simulink model "sim_lab7_disturbances"  (R2025b)
settings: Solver=ode5  StartTime=0.0  StopTime=5*T  FixedStep=1  RelTol=1e-3
model workspace (MAT data in the model file):
  Pnull = Simulink.Parameter
  Pnull.Value = Simulink.data.Expression
  Pnull.Value.ExpressionString = "zeros(3,1)"
  Pnull.Complexity = 'real'
  Pnull.Dimensions = -1
  Pnull.DataType = 'auto'
  rho_albedo_medio = Simulink.Parameter
  rho_albedo_medio.Value = 0.3
  rho_albedo_medio.Complexity = 'real'
  rho_albedo_medio.Dimensions = [1 1]
  rho_albedo_medio.DataType = 'auto'
values from neighbouring files (symbols this model uses):
  Aree = zeros(10,1)    [SCRIPT_SAD_DEMO.m]    (also in lab_7.m)
  c = astroConstants(5)*1e3    [SCRIPT_SAD_DEMO.m]    (also in lab_7.m)
  eps_E = deg2rad(astroConstants(63))    [SCRIPT_SAD_DEMO.m]    (also in lab_7.m)
  F_e = 1358    [SCRIPT_SAD_DEMO.m]    (also in lab_7.m)
  g0_1 = -29404.8e-9    (= -2.94048e-05)    [lab_7.m]
  g1_1 = -1450.9e-9    (= -1.4509e-06)    [lab_7.m]
  h1_1 = 4652.5e-9    (= 4.6525e-06)    [lab_7.m]
  j_B = [0.01; 0.05; 0.01]    [SCRIPT_SAD_DEMO.m]    (also in lab_7.m)
  J_depl = [100.9, 0, 0;           0, 25.1, 0;           0, 0, 91.6]*1e-2    [SCRIPT_SAD_DEMO.m]    (also in lab_7.m)
  kep = [a,e,incl,raan,w,theta]    [SCRIPT_SAD_DEMO.m]    (also in lab_7.m)
  mu = astroConstants(13)    [SCRIPT_SAD_DEMO.m]    (also in lab_7.m)
  n = sqrt( (mu/ (a)^3))    [SCRIPT_SAD_DEMO.m]    (also in lab_7.m = sqrt((mu/ ((a/1000)^3))))
  n_sun = 2*pi/T_sun    (= 1.99238499086e-07)    [SCRIPT_SAD_DEMO.m]    (also in lab_7.m)
  Nmat = [ ... (first row only)    [SCRIPT_SAD_DEMO.m]    (also in lab_7.m)
  r_sun = 1*ua    [SCRIPT_SAD_DEMO.m]    (also in lab_7.m)
  Re = astroConstants(23)    [SCRIPT_SAD_DEMO.m]    (also in lab_7.m)
  rf = [ ... (first row only)    [SCRIPT_SAD_DEMO.m]    (also in lab_7.m)
  rhod = 0.1*ones(10,1)    [SCRIPT_SAD_DEMO.m]    (also in lab_7.m)
  rhos = zeros(10,1)    [SCRIPT_SAD_DEMO.m]    (also in lab_7.m)
  theta = 0    [SCRIPT_SAD_DEMO.m]    (also in lab_7.m)
  w_E = deg2rad(15.04)/3600    [SCRIPT_SAD_DEMO.m]    (also in lab_7.m)
undefined symbols (not defined in the file or in its folder): SRP
libraries: LIBRARY_SAD x16, matrix_library x15
settings Model: Creator=fabio  LastModifiedBy=utente

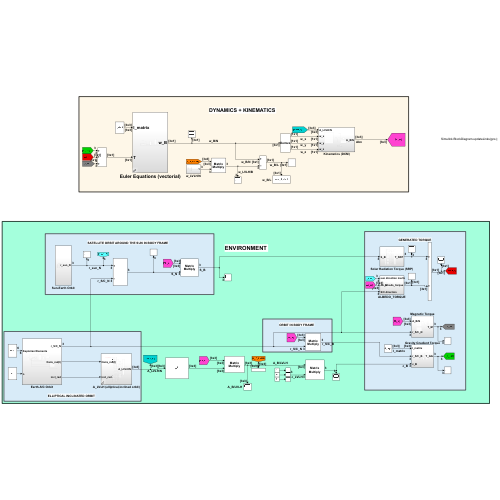
[thumbnail: Simulink's stored preview of the top-level diagram]
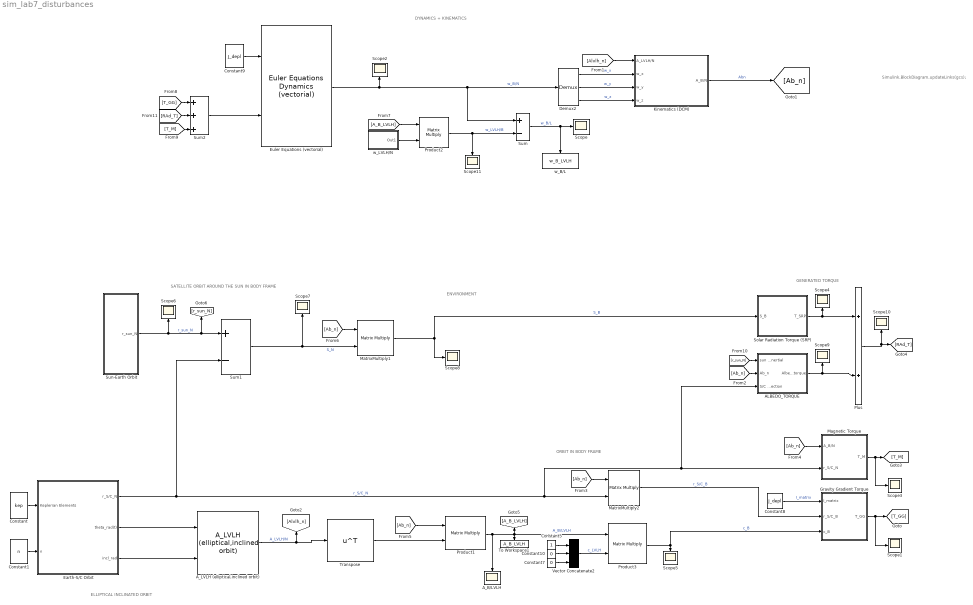
== system sim_lab7_disturbances ==
  note: Simulink.BlockDiagram.updateLinks(gcs);
  note: ORBIT IN BODY FRAME
  note: SATELLITE ORBIT AROUND THE SUN IN BODY FRAME
  note: GENERATED TORQUE
  note: ELLIPTICAL INCLINATED ORBIT
  note: ENVIRONMENT
  note: DYNAMICS + KINEMATICS
  ALBEDO_TORQUE : Subsystem
  A_B/LVLH : Scope
      settings: ActiveDisplayYMinimum=-0.55999388120508109  ActiveDisplayYMaximum=1.1733326534672313
  A_LVLH (elliptical,inclined orbit) : LIBRARY_SAD/A_LVLH (elliptical,inclined orbit)  SystemSampleTime=-1  VariantActivationTime=update diagram  EmptyChoice=off  PassThrough=off  PassThroughVariantControl=(default)  EmptyChoiceVariantControl=(default)  AllowFlexibleInterface=on  Latency=0  AutoFrameSizeCalculation=off
  Constant : Constant  Value=kep
  Constant1 : Constant  Value=n
  Constant10 : Constant  Value=0
  Constant5 : Constant
  Constant7 : Constant  Value=0
  Constant8 : Constant  Value=J_depl
  Constant9 : Constant  Value=J_depl
  Demux2 : Demux  Outputs=3
      settings: DisplayOption=none
  Earth-S/C Orbit : Subsystem
  Euler Equations (vectorial) : LIBRARY_SAD/Euler Equations Dynamics (vectorial)  SystemSampleTime=-1  VariantActivationTime=update diagram  EmptyChoice=off  PassThrough=off  PassThroughVariantControl=(default)  EmptyChoiceVariantControl=(default)  AllowFlexibleInterface=on  Latency=0  AutoFrameSizeCalculation=off
  Gravity Gradient Torque : Subsystem
  Kinematics (DCM) : Subsystem
  Magnetic Torque : Subsystem
  MatrixMultiply1 : Product  Multiplication=Matrix(*)
  MatrixMultiply2 : Product  Multiplication=Matrix(*)
  Plus : Sum
  Product1 : Product  Multiplication=Matrix(*)
  Product2 : Product  Multiplication=Matrix(*)
  Product3 : Product  Multiplication=Matrix(*)
  Scope{,1..11} (12 alike) : Scope
      Scope settings: ActiveDisplayYMinimum=-1.5011598737710617E-6  ActiveDisplayYMaximum=2.8262196534247165E-6
      Scope1 settings: DataLoggingVariableName=ScopeData3
      Scope10 settings: ActiveDisplayYMinimum=-1  ActiveDisplayYMaximum=1  DataLoggingVariableName=ScopeData27
      Scope11 settings: ActiveDisplayYMinimum=-1  ActiveDisplayYMaximum=1  DataLoggingVariableName=ScopeData21
      Scope2 settings: ActiveDisplayYMinimum=-0.00010343063306164844  ActiveDisplayYMaximum=0.00093087569755483622  DataLoggingVariableName=ScopeData2
      Scope3 settings: ActiveDisplayYMinimum=-1.6923991885641683E-6  ActiveDisplayYMaximum=1.7159675183701099E-6  DataLoggingVariableName=ScopeData4
      Scope4 settings: ActiveDisplayYMinimum=-4.3087224502121108E-24  ActiveDisplayYMaximum=4.3087224502121108E-24  DataLoggingVariableName=ScopeData16
      Scope5 settings: ActiveDisplayYMinimum=-0.55998948749949928  ActiveDisplayYMaximum=1.1733321652777222  DataLoggingVariableName=ScopeData20
      Scope6 settings: ActiveDisplayYMinimum=-1  ActiveDisplayYMaximum=1  DataLoggingVariableName=ScopeData6
      Scope7 settings: ActiveDisplayYMinimum=-1  ActiveDisplayYMaximum=1  DataLoggingVariableName=ScopeData7
      Scope8 settings: DataLoggingVariableName=ScopeData8
      Scope9 settings: ActiveDisplayYMinimum=-9.2718061255302776E-25  ActiveDisplayYMaximum=9.2718061255302776E-25  DataLoggingVariableName=ScopeData26
  Solar Radiation Torque (SRP) : Subsystem
  Sum : Sum  Inputs=+-
  Sum1 : Sum  Inputs=+-
  Sum2 : Sum  Inputs=+++
  Sun-Earth Orbit : Subsystem
  To Workspace1 : ToWorkspace  VariableName=A_B_LVLH  SampleTime=-1
  Transpose : Math  Operator=transpose
  Vector Concatenate2 : Concatenate  NumInputs=3
  w_B/L : ToWorkspace  VariableName=w_B_LVLH  SampleTime=-1
  w_LVLH/N : Subsystem
  wires:
  Euler Equations (vectorial)/1 -> Demux2/1, Sum/1, Scope2/1  "w_B/N"
  Demux2/3 -> Kinematics (DCM)/4(w_z)  "w_z"
  Product2/1 -> Scope11/1, Sum/2  "w_LVLH/B"
  Transpose/1 -> Product1/2
  Demux2/1 -> Kinematics (DCM)/2(w_x)  "w_x"
  A_LVLH (elliptical,inclined orbit)/1 -> [Alvlh_n], Transpose/1  "A_LVLH/N"
  Sum1/1 -> Scope7/1, MatrixMultiply1/2  "S_N"
  Constant/1 -> Earth-S/C Orbit/1(Keplerian Elements)
  Earth-S/C Orbit/3(incl_rad) -> A_LVLH (elliptical,inclined orbit)/2
  Product3/1 -> Gravity Gradient Torque/3(c_B), Scope5/1  "c_B"
  Constant8/1 -> Gravity Gradient Torque/1(I_matrix)  "I_matrix"
  Product1/1 -> Product3/1, [A_B_LVLH], To Workspace1/1, A_B/LVLH/1  "A_B/LVLH"
  Earth-S/C Orbit/2(theta_rad(t)) -> A_LVLH (elliptical,inclined orbit)/1
  MatrixMultiply2/1 -> Gravity Gradient Torque/2(r_S/C_B)  "r_S/C_B"
  Vector Concatenate2/1 -> Product3/2  "c_LVLH"
  Constant1/1 -> Earth-S/C Orbit/2(n)
  Constant5/1 -> Vector Concatenate2/1
  Sum2/1 -> Euler Equations (vectorial)/2
  Earth-S/C Orbit/1(r_S/C_N) -> Sum1/2, MatrixMultiply2/2, ALBEDO_TORQUE/3(S/C direction), Magnetic Torque/2(r_S/C_N)  "r_S/C_N"
  Constant10/1 -> Vector Concatenate2/2
  Constant7/1 -> Vector Concatenate2/3
  Sum/1 -> w_B/L/1, Scope/1  "w_B/L"
  Demux2/2 -> Kinematics (DCM)/3(w_y)  "w_y"
  Sun-Earth Orbit/1(r_sun_N) -> Scope6/1, Sum1/1, [r_sun_N]  "r_sun_N"
  MatrixMultiply1/1 -> Scope8/1, Solar Radiation Torque (SRP)/1(S_B)  "S_B"
  Kinematics (DCM)/1(A_B/N) -> [Ab_n]  "Abn"
  Constant9/1 -> Euler Equations (vectorial)/1
  [Ab_n] -> MatrixMultiply1/1
  [Ab_n] -> Magnetic Torque/1(A_B/N)
  [Ab_n] -> MatrixMultiply2/1
  [Ab_n] -> Product1/1
  [Alvlh_n] -> Kinematics (DCM)/1(A_LVLH/N)
  [A_B_LVLH] -> Product2/1
  Gravity Gradient Torque/1(T_GG) -> Scope1/1, [T_GG]
  Magnetic Torque/1(T_M) -> Scope3/1, [T_M]
  Solar Radiation Torque (SRP)/1(T_SRP) -> Plus/1, Scope4/1
  [RAd_T] -> Sum2/2
  [T_GG] -> Sum2/1
  [T_M] -> Sum2/3
  w_LVLH/N/1(Out1) -> Product2/2
  [r_sun_N] -> ALBEDO_TORQUE/1(sun direction inertial)
  [Ab_n] -> ALBEDO_TORQUE/2(Ab_n)
  ALBEDO_TORQUE/1(Albedo_torque) -> Scope9/1, Plus/2
  Plus/1 -> Scope10/1, [RAd_T]

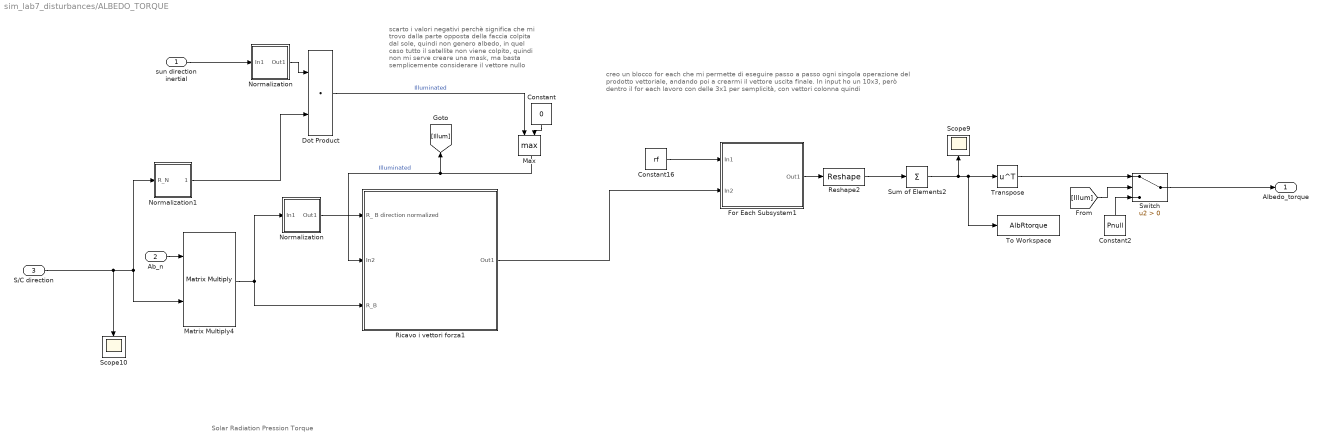
== system sim_lab7_disturbances/ALBEDO_TORQUE ==
  note: Solar Radiation Pression Torque
  note: creo un blocco for each che mi permette di eseguire passo a passo ogni singola operazione del prodotto vettoriale, andando poi a crearmi il vettore uscita finale. In input ho un 10x3, però dentro il for each lavoro con delle 3x1 per semplicità, con vettori colonna quindi
  note: scarto i valori negativi perchè significa che mi trovo dalla parte opposta della faccia colpita dal sole, quindi non genero albedo, in quel caso tutto il satellite non viene colpito, quindi non mi serve creare una mask, ma basta semplicemente considerare il vettore nullo
  sun direction inertial : Inport
  Ab_n : Inport  Port=2
  S/C direction : Inport  Port=3
  Constant : Constant  Value=0
  Constant16 : Constant  Value=rf
  Constant2 : Constant  Value=Pnull
  Dot Product : DotProduct  OutDataTypeStr=Inherit: Inherit via internal rule
  For Each Subsystem1 : Subsystem  TreatAsAtomicUnit=on
  Matrix Multiply4 : Product  Multiplication=Matrix(*)
  Max : MinMax  Function=max  Inputs=2
  Normalization : Subsystem
  "Normalization " : Subsystem
  Normalization1 : Subsystem
  Reshape2 : Reshape  OutputDimensionality=Customize  OutputDimensions=[10 3]
  Ricavo i vettori forza1 : Subsystem
  Scope10 : Scope
      settings: ActiveDisplayYMinimum=-8805.2567998384475  ActiveDisplayYMaximum=8127.929464306656  DataLoggingVariableName=ScopeData17
  Scope9 : Scope
      settings: ActiveDisplayYMinimum=-9.2718061255302776E-25  ActiveDisplayYMaximum=2.6543612251060555E-24  DataLoggingVariableName=ScopeData25
  Sum of Elements2 : Sum  Inputs=+  CollapseMode=Specified dimension
  Switch : Switch  Criteria=u2 > Threshold  SaturateOnIntegerOverflow=off  InputSameDT=off
  To Workspace : ToWorkspace  VariableName=AlbRtorque  SampleTime=-1
  Transpose : Math  Operator=transpose
  Albedo_torque : Outport
  wires:
  Sum of Elements2/1 -> Transpose/1, To Workspace/1, Scope9/1
  Matrix Multiply4/1 -> Normalization/1(In1), Ricavo i vettori forza1/3(R_B)
  Normalization1/1(Out1) -> Dot Product/2
  Ricavo i vettori forza1/1(Out1) -> For Each Subsystem1/2(In2)
  For Each Subsystem1/1(Out1) -> Reshape2/1
  S/C direction/1 -> Scope10/1, Matrix Multiply4/2, Normalization1/1(R_N)
  "Normalization "/1(Out1) -> Dot Product/1
  Constant16/1 -> For Each Subsystem1/1(In1)
  Normalization/1(Out1) -> Ricavo i vettori forza1/1(" R_ B direction normalized")
  Dot Product/1 -> Max/1  "Illuminated"
  Ab_n/1 -> Matrix Multiply4/1
  sun direction inertial/1 -> "Normalization "/1(In1)
  Constant2/1 -> Switch/3
  Reshape2/1 -> Sum of Elements2/1
  Constant/1 -> Max/2
  Transpose/1 -> Switch/1
  Switch/1 -> Albedo_torque/1
  Max/1 -> Ricavo i vettori forza1/2(In2), [Illum]  "Illuminated"
  [Illum] -> Switch/2

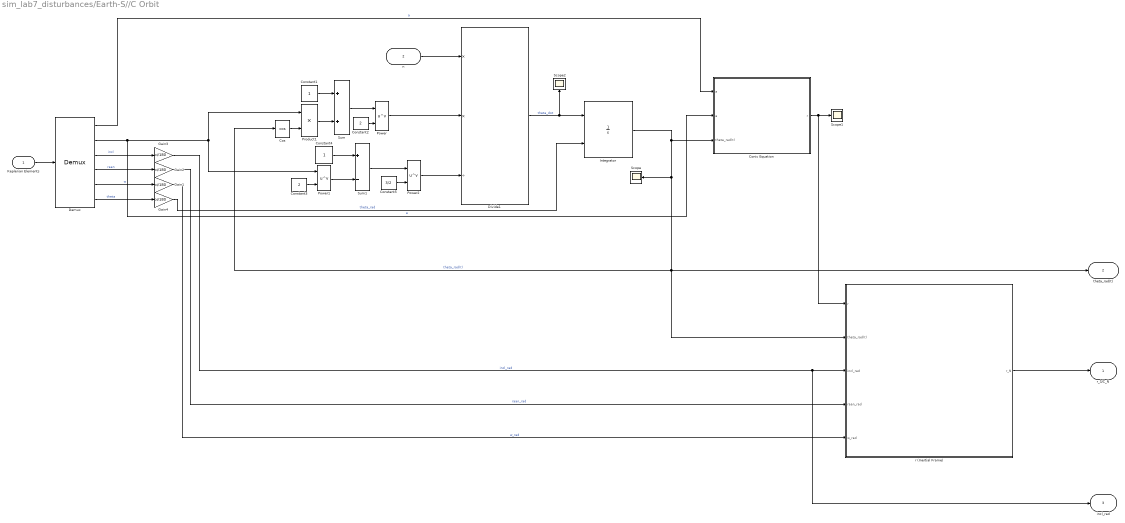
== system sim_lab7_disturbances/Earth-S//C Orbit ==
  Keplerian Elements : Inport
  n : Inport  Port=2
  Conic Equation : Subsystem
  Constant1 : Constant
  Constant2 : Constant  Value=2
  Constant3 : Constant  Value=2
  Constant4 : Constant
  Constant5 : Constant  Value=3/2
  Cos : Trigonometry  Operator=cos
  Demux : Demux  Outputs=6
      settings: DisplayOption=none
  Divide1 : Product  Inputs=**/
  Gain{1..4} (4 alike) : Gain  Gain=pi/180
  Integrator : Integrator  InitialConditionSource=external  InitialCondition=theta  WrapState=on  WrappedStateUpperValue=2*pi  WrappedStateLowerValue=0
  Power : Math  Operator=pow
  Power1 : Math  Operator=pow
  Power2 : Math  Operator=pow
  Product1 : Product
  Scope : Scope
      settings: ActiveDisplayYMinimum=-0.785387370168924  ActiveDisplayYMaximum=7.0684863315203179  DataLoggingVariableName=ScopeData22
  Scope1 : Scope
      settings: ActiveDisplayYMinimum=6287.5500000061184  ActiveDisplayYMaximum=10412.44999994494  DataLoggingVariableName=ScopeData23
  Scope2 : Scope
      settings: ActiveDisplayYMinimum=0.00072744506449318766  ActiveDisplayYMaximum=0.00092744506449318775  DataLoggingVariableName=ScopeData24
  Sum : Sum
  Sum1 : Sum  Inputs=+-
  r (Inertial Frame) : Subsystem
  r_S/C_N : Outport
  theta_rad(t) : Outport  Port=2
  incl_rad : Outport  Port=3
  wires:
  Keplerian Elements/1 -> Demux/1
  Demux/1 -> Conic Equation/1(a)  "a"
  Demux/2 -> Conic Equation/2(e), Product1/1, Power1/1  "e"
  Demux/3 -> Gain3/1  "incl"
  Demux/4 -> Gain2/1  "raan"
  Demux/5 -> Gain1/1  "w"
  Demux/6 -> Gain4/1  "theta"
  Constant1/1 -> Sum/1
  Cos/1 -> Product1/2
  Product1/1 -> Sum/2
  Sum/1 -> Power/1
  Constant2/1 -> Power/2
  Power/1 -> Divide1/2
  Constant3/1 -> Power1/2
  Power1/1 -> Sum1/2
  Constant4/1 -> Sum1/1
  Constant5/1 -> Power2/2
  Sum1/1 -> Power2/1
  Power2/1 -> Divide1/3
  Divide1/1 -> Scope2/1, Integrator/1  "theta_dot"
  Integrator/1 -> Scope/1, Cos/1, r (Inertial Frame)/2(theta_rad(t)), theta_rad(t)/1, Conic Equation/3(theta_rad(t))  "theta_rad(t)"
  Conic Equation/1(r) -> r (Inertial Frame)/1(r), Scope1/1
  Gain3/1 -> incl_rad/1, r (Inertial Frame)/3(incl_rad)  "incl_rad"
  Gain2/1 -> r (Inertial Frame)/4(raan_rad)  "raan_rad"
  Gain1/1 -> r (Inertial Frame)/5(w_rad)  "w_rad"
  r (Inertial Frame)/1(r_N) -> r_S/C_N/1
  n/1 -> Divide1/1
  Gain4/1 -> Integrator/2  "theta_rad"

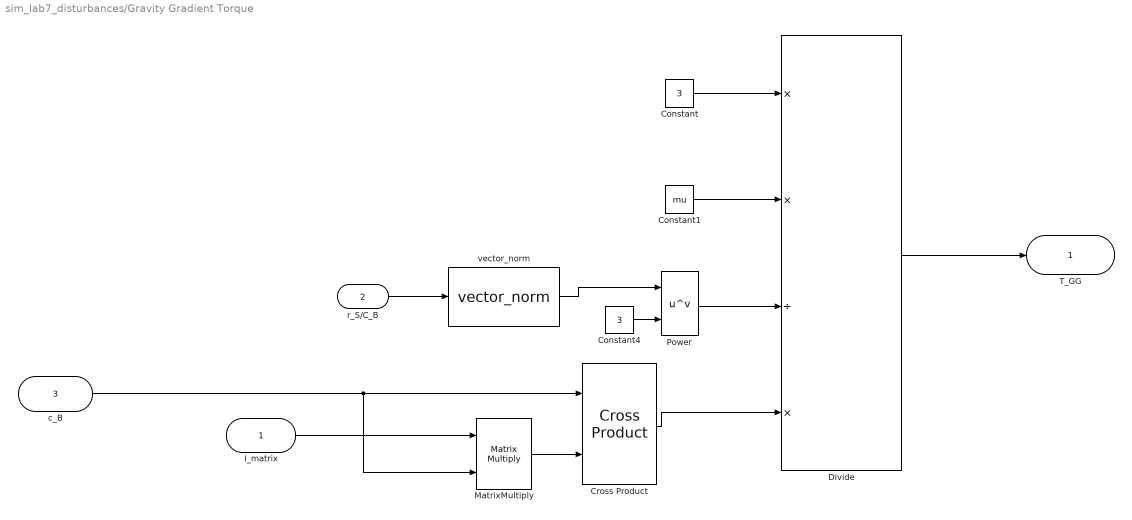
== system sim_lab7_disturbances/Gravity Gradient Torque ==
  I_matrix : Inport
  r_S/C_B : Inport  Port=2
  c_B : Inport  Port=3
  Constant : Constant  Value=3
  Constant1 : Constant  Value=mu
  Constant4 : Constant  Value=3
  Cross Product : matrix_library/Cross Product
  Divide : Product  Inputs=**/*
  MatrixMultiply : Product  Multiplication=Matrix(*)
  Power : Math  Operator=pow
  vector_norm : LIBRARY_SAD/vector_norm  SystemSampleTime=-1  VariantActivationTime=update diagram  EmptyChoice=off  PassThrough=off  PassThroughVariantControl=(default)  EmptyChoiceVariantControl=(default)  AllowFlexibleInterface=on  Latency=0  AutoFrameSizeCalculation=off
  T_GG : Outport
  wires:
  r_S/C_B/1 -> vector_norm/1
  Constant4/1 -> Power/2
  Constant/1 -> Divide/1
  Constant1/1 -> Divide/2
  Power/1 -> Divide/3
  I_matrix/1 -> MatrixMultiply/1
  c_B/1 -> MatrixMultiply/2, Cross Product/1
  MatrixMultiply/1 -> Cross Product/2
  Cross Product/1 -> Divide/4
  Divide/1 -> T_GG/1
  vector_norm/1 -> Power/1

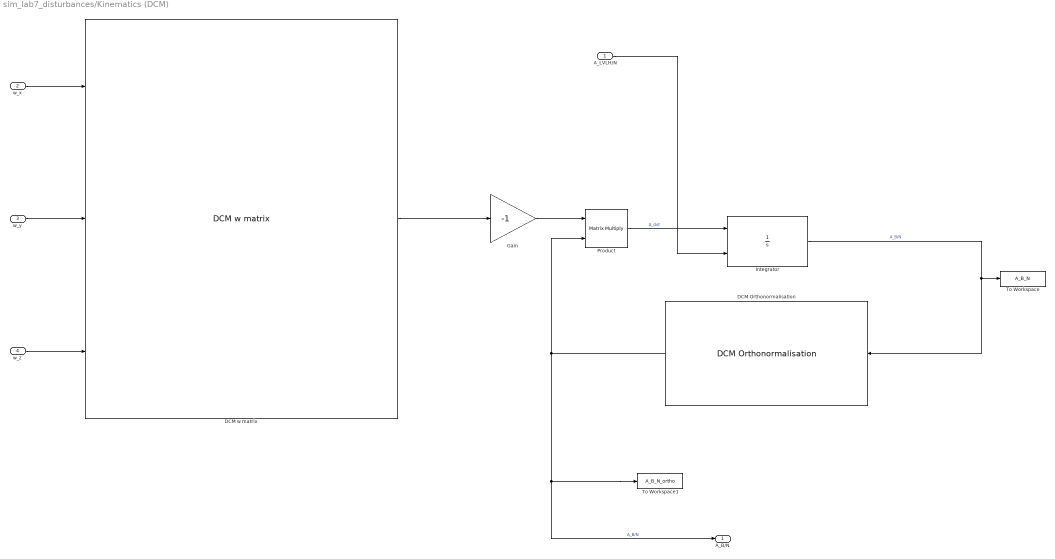
== system sim_lab7_disturbances/Kinematics (DCM) ==
  A_LVLH/N : Inport
  w_x : Inport  Port=2
  w_y : Inport  Port=3
  w_z : Inport  Port=4
  DCM Orthonormalisation : LIBRARY_SAD/DCM Orthonormalisation  SystemSampleTime=-1  VariantActivationTime=update diagram  EmptyChoice=off  PassThrough=off  PassThroughVariantControl=(default)  EmptyChoiceVariantControl=(default)  AllowFlexibleInterface=on  Latency=0  AutoFrameSizeCalculation=off
  DCM w matrix : LIBRARY_SAD/DCM w matrix  SystemSampleTime=-1  VariantActivationTime=update diagram  EmptyChoice=off  PassThrough=off  PassThroughVariantControl=(default)  EmptyChoiceVariantControl=(default)  AllowFlexibleInterface=on  Latency=0  AutoFrameSizeCalculation=off
  Gain : Gain  Gain=-1
  Integrator : Integrator  InitialConditionSource=external
  Product : Product  Multiplication=Matrix(*)
  To Workspace : ToWorkspace  VariableName=A_B_N  SampleTime=-1
  To Workspace1 : ToWorkspace  VariableName=A_B_N_ortho  SampleTime=-1
  A_B/N : Outport
  wires:
  A_LVLH/N/1 -> Integrator/2
  w_y/1 -> DCM w matrix/2
  w_z/1 -> DCM w matrix/3
  Integrator/1 -> To Workspace/1, DCM Orthonormalisation/1  "A_B/N"
  Product/1 -> Integrator/1  "A_dot"
  DCM w matrix/1 -> Gain/1
  w_x/1 -> DCM w matrix/1
  Gain/1 -> Product/1
  DCM Orthonormalisation/1 -> To Workspace1/1, A_B/N/1, Product/2  "A_B/N"

== system sim_lab7_disturbances/Magnetic Torque ==
  A_B/N : Inport
  r_S/C_N : Inport  Port=2
  B_N (IGRF Gauss Model - Order N) : Subsystem  Commented=on
  B_N (Simple Dipole Model) : Subsystem
  Constant : Constant  Value=j_B
  Cross Product : matrix_library/Cross Product
  MatrixMultiply : Product  Multiplication=Matrix(*)
  Scope : Scope
      settings: ActiveDisplayYMinimum=-1  ActiveDisplayYMaximum=1  DataLoggingVariableName=ScopeData5
  T_M : Outport
  wires:
  r_S/C_N/1 -> B_N (Simple Dipole Model)/1(r_S/C_N)
  B_N (Simple Dipole Model)/1(B_N) -> MatrixMultiply/2
  A_B/N/1 -> MatrixMultiply/1
  MatrixMultiply/1 -> Scope/1, Cross Product/2  "B_B"
  Constant/1 -> Cross Product/1
  Cross Product/1 -> T_M/1

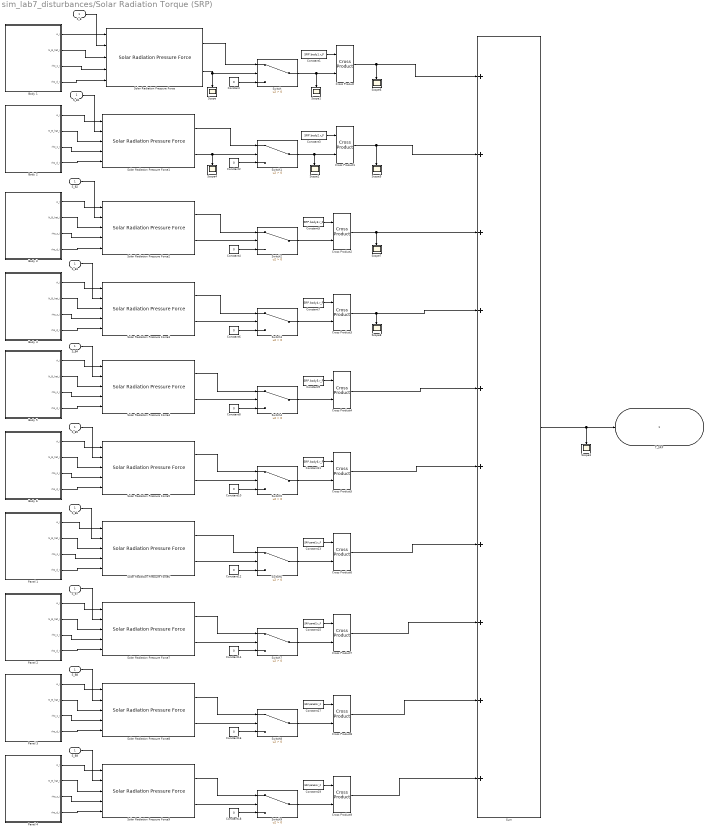
== system sim_lab7_disturbances/Solar Radiation Torque (SRP) ==
  S_B : Inport
  Body 1 : Subsystem
  Body 2 : Subsystem
  Body 3 : Subsystem
  Body 4 : Subsystem
  Body 5 : Subsystem
  Body 6 : Subsystem
  Constant{,2,4,6,8,10,12,14,16,18} (10 alike) : Constant  Value=0
  Constant1 : Constant  Value=SRP.body1.r_F
  Constant11 : Constant  Value=SRP.body6.r_F
  Constant13 : Constant  Value=SRP.panel1.r_F
  Constant15 : Constant  Value=SRP.panel2.r_F
  Constant17 : Constant  Value=SRP.panel3.r_F
  Constant19 : Constant  Value=SRP.panel4.r_F
  Constant3 : Constant  Value=SRP.body2.r_F
  Constant5 : Constant  Value=SRP.body3.r_F
  Constant7 : Constant  Value=SRP.body4.r_F
  Constant9 : Constant  Value=SRP.body5.r_F
  Cross Product{,1..9} (10 alike) : matrix_library/Cross Product
  Panel 1 : Subsystem
  Panel 2 : Subsystem
  Panel 3 : Subsystem
  Panel 4 : Subsystem
  S_B{1..9} (9 alike) : InportShadow
  Scope{,1..8} (9 alike) : Scope
      Scope settings: ActiveDisplayYMinimum=-1  ActiveDisplayYMaximum=1  DataLoggingVariableName=ScopeData9
      Scope1 settings: ActiveDisplayYMinimum=-1  ActiveDisplayYMaximum=1  DataLoggingVariableName=ScopeData10
      Scope2 settings: ActiveDisplayYMinimum=-1  ActiveDisplayYMaximum=1  DataLoggingVariableName=ScopeData11
      Scope3 settings: ActiveDisplayYMinimum=-5.1359030627651383E-25  ActiveDisplayYMaximum=9.2718061255302776E-25  DataLoggingVariableName=ScopeData12
      Scope4 settings: ActiveDisplayYMinimum=-1  ActiveDisplayYMaximum=1  DataLoggingVariableName=ScopeData13
      Scope5 settings: ActiveDisplayYMinimum=-1  ActiveDisplayYMaximum=1  DataLoggingVariableName=ScopeData14
      Scope6 settings: ActiveDisplayYMinimum=-1  ActiveDisplayYMaximum=1  DataLoggingVariableName=ScopeData15
      Scope7 settings: ActiveDisplayYMinimum=-1  ActiveDisplayYMaximum=1  DataLoggingVariableName=ScopeData18
      Scope8 settings: ActiveDisplayYMinimum=-1  ActiveDisplayYMaximum=1  DataLoggingVariableName=ScopeData19
  Solar Radiation Pressure Force : LIBRARY_SAD/Solar Radiation Pressure Force  SystemSampleTime=-1  VariantActivationTime=update diagram  EmptyChoice=off  PassThrough=off  PassThroughVariantControl=(default)  EmptyChoiceVariantControl=(default)  AllowFlexibleInterface=on  Latency=0  AutoFrameSizeCalculation=off
      link override vector_norm: SourceBlock=LIBRARY_SAD/vector_norm
  Solar Radiation Pressure Force1 : LIBRARY_SAD/Solar Radiation Pressure Force  SystemSampleTime=-1  VariantActivationTime=update diagram  EmptyChoice=off  PassThrough=off  PassThroughVariantControl=(default)  EmptyChoiceVariantControl=(default)  AllowFlexibleInterface=on  Latency=0  AutoFrameSizeCalculation=off
      link override vector_norm: SourceBlock=LIBRARY_SAD/vector_norm
  Solar Radiation Pressure Force2 : LIBRARY_SAD/Solar Radiation Pressure Force  SystemSampleTime=-1  VariantActivationTime=update diagram  EmptyChoice=off  PassThrough=off  PassThroughVariantControl=(default)  EmptyChoiceVariantControl=(default)  AllowFlexibleInterface=on  Latency=0  AutoFrameSizeCalculation=off
      link override vector_norm: SourceBlock=LIBRARY_SAD/vector_norm
  Solar Radiation Pressure Force3 : LIBRARY_SAD/Solar Radiation Pressure Force  SystemSampleTime=-1  VariantActivationTime=update diagram  EmptyChoice=off  PassThrough=off  PassThroughVariantControl=(default)  EmptyChoiceVariantControl=(default)  AllowFlexibleInterface=on  Latency=0  AutoFrameSizeCalculation=off
      link override vector_norm: SourceBlock=LIBRARY_SAD/vector_norm
  Solar Radiation Pressure Force4 : LIBRARY_SAD/Solar Radiation Pressure Force  SystemSampleTime=-1  VariantActivationTime=update diagram  EmptyChoice=off  PassThrough=off  PassThroughVariantControl=(default)  EmptyChoiceVariantControl=(default)  AllowFlexibleInterface=on  Latency=0  AutoFrameSizeCalculation=off
      link override vector_norm: SourceBlock=LIBRARY_SAD/vector_norm
  Solar Radiation Pressure Force5 : LIBRARY_SAD/Solar Radiation Pressure Force  SystemSampleTime=-1  VariantActivationTime=update diagram  EmptyChoice=off  PassThrough=off  PassThroughVariantControl=(default)  EmptyChoiceVariantControl=(default)  AllowFlexibleInterface=on  Latency=0  AutoFrameSizeCalculation=off
      link override vector_norm: SourceBlock=LIBRARY_SAD/vector_norm
  Solar Radiation Pressure Force6 : LIBRARY_SAD/Solar Radiation Pressure Force  SystemSampleTime=-1  VariantActivationTime=update diagram  EmptyChoice=off  PassThrough=off  PassThroughVariantControl=(default)  EmptyChoiceVariantControl=(default)  AllowFlexibleInterface=on  Latency=0  AutoFrameSizeCalculation=off
      link override vector_norm: SourceBlock=LIBRARY_SAD/vector_norm
  Solar Radiation Pressure Force7 : LIBRARY_SAD/Solar Radiation Pressure Force  SystemSampleTime=-1  VariantActivationTime=update diagram  EmptyChoice=off  PassThrough=off  PassThroughVariantControl=(default)  EmptyChoiceVariantControl=(default)  AllowFlexibleInterface=on  Latency=0  AutoFrameSizeCalculation=off
      link override vector_norm: SourceBlock=LIBRARY_SAD/vector_norm
  Solar Radiation Pressure Force8 : LIBRARY_SAD/Solar Radiation Pressure Force  SystemSampleTime=-1  VariantActivationTime=update diagram  EmptyChoice=off  PassThrough=off  PassThroughVariantControl=(default)  EmptyChoiceVariantControl=(default)  AllowFlexibleInterface=on  Latency=0  AutoFrameSizeCalculation=off
      link override vector_norm: SourceBlock=LIBRARY_SAD/vector_norm
  Solar Radiation Pressure Force9 : LIBRARY_SAD/Solar Radiation Pressure Force  SystemSampleTime=-1  VariantActivationTime=update diagram  EmptyChoice=off  PassThrough=off  PassThroughVariantControl=(default)  EmptyChoiceVariantControl=(default)  AllowFlexibleInterface=on  Latency=0  AutoFrameSizeCalculation=off
      link override vector_norm: SourceBlock=LIBRARY_SAD/vector_norm
  Sum : Sum  Inputs=++++++++++
  Switch{,1..9} (10 alike) : Switch  Criteria=u2 > Threshold  SaturateOnIntegerOverflow=off  InputSameDT=off
  T_SRP : Outport
  wires:
  S_B/1 -> Solar Radiation Pressure Force/2
  Body 1/1(A_i) -> Solar Radiation Pressure Force/1
  Body 1/2(N_B_hat_i) -> Solar Radiation Pressure Force/3
  Body 1/3(rho_s_i) -> Solar Radiation Pressure Force/4
  Body 1/4(rho_d_i) -> Solar Radiation Pressure Force/5
  Solar Radiation Pressure Force/1 -> Switch/1
  Solar Radiation Pressure Force/2 -> Scope/1, Switch/2
  Body 2/4(rho_d_i) -> Solar Radiation Pressure Force1/5
  Body 2/3(rho_s_i) -> Solar Radiation Pressure Force1/4
  Body 2/2(N_B_hat_i) -> Solar Radiation Pressure Force1/3
  Body 2/1(A_i) -> Solar Radiation Pressure Force1/1
  S_B1/1 -> Solar Radiation Pressure Force1/2
  S_B2/1 -> Solar Radiation Pressure Force2/2
  Body 3/1(A_i) -> Solar Radiation Pressure Force2/1
  Body 3/2(N_B_hat_i) -> Solar Radiation Pressure Force2/3
  Body 3/3(rho_s_i) -> Solar Radiation Pressure Force2/4
  Body 3/4(rho_d_i) -> Solar Radiation Pressure Force2/5
  Body 4/4(rho_d_i) -> Solar Radiation Pressure Force3/5
  Body 4/3(rho_s_i) -> Solar Radiation Pressure Force3/4
  Body 4/2(N_B_hat_i) -> Solar Radiation Pressure Force3/3
  Body 4/1(A_i) -> Solar Radiation Pressure Force3/1
  S_B3/1 -> Solar Radiation Pressure Force3/2
  S_B4/1 -> Solar Radiation Pressure Force4/2
  Body 5/1(A_i) -> Solar Radiation Pressure Force4/1
  Body 5/2(N_B_hat_i) -> Solar Radiation Pressure Force4/3
  Body 5/3(rho_s_i) -> Solar Radiation Pressure Force4/4
  Body 5/4(rho_d_i) -> Solar Radiation Pressure Force4/5
  Body 6/4(rho_d_i) -> Solar Radiation Pressure Force5/5
  Body 6/3(rho_s_i) -> Solar Radiation Pressure Force5/4
  Body 6/2(N_B_hat_i) -> Solar Radiation Pressure Force5/3
  Body 6/1(A_i) -> Solar Radiation Pressure Force5/1
  S_B5/1 -> Solar Radiation Pressure Force5/2
  S_B6/1 -> Solar Radiation Pressure Force6/2
  Panel 1/1(A_i) -> Solar Radiation Pressure Force6/1
  Panel 1/2(N_B_hat_i) -> Solar Radiation Pressure Force6/3
  Panel 1/3(rho_s_i) -> Solar Radiation Pressure Force6/4
  Panel 1/4(rho_d_i) -> Solar Radiation Pressure Force6/5
  Panel 2/4(rho_d_i) -> Solar Radiation Pressure Force7/5
  Panel 2/3(rho_s_i) -> Solar Radiation Pressure Force7/4
  Panel 2/2(N_B_hat_i) -> Solar Radiation Pressure Force7/3
  Panel 2/1(A_i) -> Solar Radiation Pressure Force7/1
  S_B7/1 -> Solar Radiation Pressure Force7/2
  S_B8/1 -> Solar Radiation Pressure Force8/2
  Panel 3/1(A_i) -> Solar Radiation Pressure Force8/1
  Panel 3/2(N_B_hat_i) -> Solar Radiation Pressure Force8/3
  Panel 3/3(rho_s_i) -> Solar Radiation Pressure Force8/4
  Panel 3/4(rho_d_i) -> Solar Radiation Pressure Force8/5
  Panel 4/4(rho_d_i) -> Solar Radiation Pressure Force9/5
  Panel 4/3(rho_s_i) -> Solar Radiation Pressure Force9/4
  Panel 4/2(N_B_hat_i) -> Solar Radiation Pressure Force9/3
  Panel 4/1(A_i) -> Solar Radiation Pressure Force9/1
  S_B9/1 -> Solar Radiation Pressure Force9/2
  Constant/1 -> Switch/3
  Switch/1 -> Scope1/1, Cross Product/2
  Constant1/1 -> Cross Product/1
  Cross Product/1 -> Scope6/1, Sum/1
  Cross Product1/1 -> Sum/2, Scope5/1
  Constant3/1 -> Cross Product1/1
  Switch1/1 -> Scope2/1, Cross Product1/2
  Constant2/1 -> Switch1/3
  Solar Radiation Pressure Force1/2 -> Scope4/1, Switch1/2
  Solar Radiation Pressure Force1/1 -> Switch1/1
  Solar Radiation Pressure Force2/1 -> Switch2/1
  Solar Radiation Pressure Force2/2 -> Switch2/2
  Constant4/1 -> Switch2/3
  Switch2/1 -> Cross Product2/2
  Constant5/1 -> Cross Product2/1
  Cross Product2/1 -> Scope7/1, Sum/3
  Cross Product3/1 -> Scope8/1, Sum/4
  Constant7/1 -> Cross Product3/1
  Switch3/1 -> Cross Product3/2
  Constant6/1 -> Switch3/3
  Solar Radiation Pressure Force3/2 -> Switch3/2
  Solar Radiation Pressure Force3/1 -> Switch3/1
  Solar Radiation Pressure Force4/1 -> Switch4/1
  Solar Radiation Pressure Force4/2 -> Switch4/2
  Constant8/1 -> Switch4/3
  Switch4/1 -> Cross Product4/2
  Constant9/1 -> Cross Product4/1
  Cross Product4/1 -> Sum/5
  Cross Product5/1 -> Sum/6
  Constant11/1 -> Cross Product5/1
  Switch5/1 -> Cross Product5/2
  Constant10/1 -> Switch5/3
  Solar Radiation Pressure Force5/2 -> Switch5/2
  Solar Radiation Pressure Force5/1 -> Switch5/1
  Solar Radiation Pressure Force6/1 -> Switch6/1
  Solar Radiation Pressure Force6/2 -> Switch6/2
  Constant12/1 -> Switch6/3
  Switch6/1 -> Cross Product6/2
  Constant13/1 -> Cross Product6/1
  Cross Product6/1 -> Sum/7
  Cross Product7/1 -> Sum/8
  Constant15/1 -> Cross Product7/1
  Switch7/1 -> Cross Product7/2
  Constant14/1 -> Switch7/3
  Solar Radiation Pressure Force7/2 -> Switch7/2
  Solar Radiation Pressure Force7/1 -> Switch7/1
  Solar Radiation Pressure Force8/1 -> Switch8/1
  Solar Radiation Pressure Force8/2 -> Switch8/2
  Constant16/1 -> Switch8/3
  Switch8/1 -> Cross Product8/2
  Constant17/1 -> Cross Product8/1
  Cross Product8/1 -> Sum/9
  Cross Product9/1 -> Sum/10
  Constant19/1 -> Cross Product9/1
  Switch9/1 -> Cross Product9/2
  Constant18/1 -> Switch9/3
  Solar Radiation Pressure Force9/2 -> Switch9/2
  Solar Radiation Pressure Force9/1 -> Switch9/1
  Sum/1 -> Scope3/1, T_SRP/1

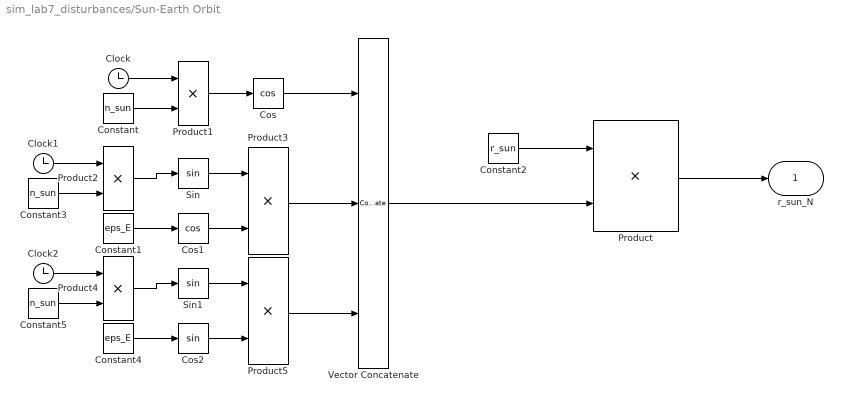
== system sim_lab7_disturbances/Sun-Earth Orbit ==
  Clock : Clock
  Clock1 : Clock
  Clock2 : Clock
  Constant : Constant  Value=n_sun
  Constant1 : Constant  Value=eps_E
  Constant2 : Constant  Value=r_sun
  Constant3 : Constant  Value=n_sun
  Constant4 : Constant  Value=eps_E
  Constant5 : Constant  Value=n_sun
  Cos : Trigonometry  Operator=cos
  Cos1 : Trigonometry  Operator=cos
  Cos2 : Trigonometry
  Product{,1..5} (6 alike) : Product
  Sin : Trigonometry
  Sin1 : Trigonometry
  Vector Concatenate : Concatenate  NumInputs=3
  r_sun_N : Outport
  wires:
  Constant2/1 -> Product/1
  Clock/1 -> Product1/1
  Constant/1 -> Product1/2
  Product1/1 -> Cos/1
  Cos/1 -> Vector Concatenate/1
  Product2/1 -> Sin/1
  Constant3/1 -> Product2/2
  Clock1/1 -> Product2/1
  Sin/1 -> Product3/1
  Constant1/1 -> Cos1/1
  Product3/1 -> Vector Concatenate/2
  Cos1/1 -> Product3/2
  Cos2/1 -> Product5/2
  Product5/1 -> Vector Concatenate/3
  Constant4/1 -> Cos2/1
  Sin1/1 -> Product5/1
  Clock2/1 -> Product4/1
  Constant5/1 -> Product4/2
  Product4/1 -> Sin1/1
  Vector Concatenate/1 -> Product/2
  Product/1 -> r_sun_N/1

== system sim_lab7_disturbances/w_LVLH//N ==
  Constant2 : Constant  Value=0
  Constant3 : Constant  Value=0
  Constant4 : Constant  Value=n
  Vector Concatenate1 : Concatenate  NumInputs=3
  Out1 : Outport
  wires:
  Vector Concatenate1/1 -> Out1/1  "w_LVLH/N"
  Constant2/1 -> Vector Concatenate1/1
  Constant3/1 -> Vector Concatenate1/2
  Constant4/1 -> Vector Concatenate1/3

== system sim_lab7_disturbances/ALBEDO_TORQUE/For Each Subsystem1 ==
  note: nelle proprietà lascio direttamente così almeno posso processare una alla volta le singole righe e colonne sia in dimension che in width
  In1 : Inport  Partition=on  PartitionDimension=1  PartitionWidth=1  PartitionOffset=0
  In2 : Inport  Port=2  Partition=on  PartitionDimension=1  PartitionWidth=1  PartitionOffset=0
  Cross Product : matrix_library/Cross Product
  For Each : ForEach  DisableCoverage=on
  Signal Specification : SignalSpecification  Dimensions=[1 3]
  Transpose : Math  Operator=transpose
  Transpose1 : Math  Operator=transpose
  Transpose2 : Math  Operator=transpose
  Out1 : Outport  ConcatenationDimension=1
  wires:
  In2/1 -> Transpose/1  "Rfi"
  In1/1 -> Transpose1/1  "Fi"
  Transpose/1 -> Cross Product/1
  Transpose1/1 -> Cross Product/2
  Cross Product/1 -> Transpose2/1
  Transpose2/1 -> Signal Specification/1
  Signal Specification/1 -> Out1/1

== system sim_lab7_disturbances/ALBEDO_TORQUE/Normalization ==
  In1 : Inport
  Divide : Product  Inputs=*/
  Dot Product : DotProduct  OutDataTypeStr=Inherit: Inherit via internal rule
  Sqrt : Sqrt
  Out1 : Outport
  wires:
  Dot Product/1 -> Sqrt/1
  In1/1 -> Divide/1, Dot Product/2, Dot Product/1
  Divide/1 -> Out1/1
  Sqrt/1 -> Divide/2

== system sim_lab7_disturbances/ALBEDO_TORQUE/Normalization  ==
  In1 : Inport
  Divide : Product  Inputs=*/
  Dot Product : DotProduct  OutDataTypeStr=Inherit: Inherit via internal rule
  Sqrt : Sqrt
  Out1 : Outport
  wires:
  Dot Product/1 -> Sqrt/1
  In1/1 -> Divide/1, Dot Product/2, Dot Product/1
  Divide/1 -> Out1/1
  Sqrt/1 -> Divide/2

== system sim_lab7_disturbances/ALBEDO_TORQUE/Normalization1 ==
  R_N : Inport
  Divide : Product  Inputs=*/
  Dot Product : DotProduct  OutDataTypeStr=Inherit: Inherit via internal rule
  Sqrt : Sqrt
  Out1 : Outport
  wires:
  Dot Product/1 -> Sqrt/1
  R_N/1 -> Divide/1, Dot Product/2, Dot Product/1
  Divide/1 -> Out1/1
  Sqrt/1 -> Divide/2

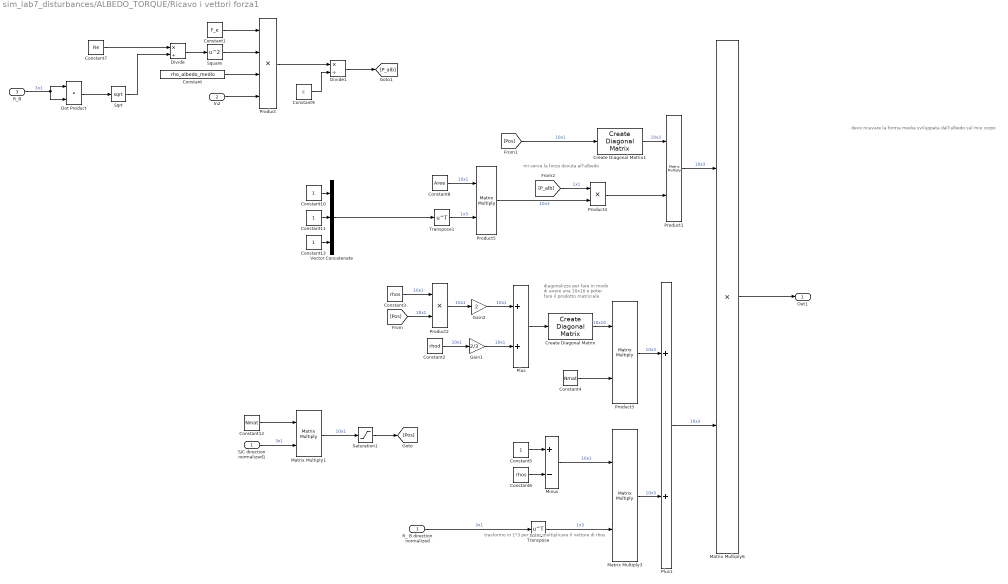
== system sim_lab7_disturbances/ALBEDO_TORQUE/Ricavo i vettori forza1 ==
  note: devo ricavare la forma media sviluppata dall'albedo sul mio corpo
  note: mi serve la forza dovuta all'albedo
  note: diagonalizzo per fare in modo di avere una 10x10 e poter fare il prodotto matriciale
  note: trasformo in 1*3 per poter moltiplicare il vettore di rhos
  " R_ B direction normalized" : Inport
  In2 : Inport  Port=2
  R_B : Inport  Port=3
  Constant : Constant  Value=rho_albedo_medio
  Constant1 : Constant  Value=F_e
  Constant{5,10..11,13} (4 alike) : Constant
  Constant12 : Constant  Value=Nmat
  Constant2 : Constant  Value=rhod
  Constant3 : Constant  Value=rhos
  Constant4 : Constant  Value=Nmat
  Constant6 : Constant  Value=rhos
  Constant7 : Constant  Value=Re
  Constant8 : Constant  Value=Aree
  Constant9 : Constant  Value=c
  Create Diagonal Matrix : matrix_library/Create Diagonal Matrix
      settings: LibrarySourceBlock=|
      | simulink/Matrix
      | Operations/Create Diagonal
      | Matrix
  Create Diagonal Matrix1 : matrix_library/Create Diagonal Matrix
      settings: LibrarySourceBlock=|
      | simulink/Matrix
      | Operations/Create Diagonal
      | Matrix
  Divide : Product  Inputs=*/
  Divide1 : Product  Inputs=*/
  Dot Product : DotProduct  OutDataTypeStr=Inherit: Inherit via internal rule
  Gain1 : Gain  Gain=2/3
  Gain2 : Gain  Gain=2
  Matrix Multiply1 : Product  Multiplication=Matrix(*)
  Matrix Multiply3 : Product  Multiplication=Matrix(*)
  Matrix Multiply6 : Product
  Minus : Sum  Inputs=+-
  Plus : Sum
  Plus1 : Sum
  Product : Product  Inputs=4
  Product1 : Product  Multiplication=Matrix(*)
  Product2 : Product
  Product3 : Product  Multiplication=Matrix(*)
  Product4 : Product
  Product5 : Product  Multiplication=Matrix(*)
  S/C direction normalized1 : InportShadow
  Saturation1 : Saturate  UpperLimit=inf  LowerLimit=0
  Sqrt : Sqrt
  Square : Math  Operator=square
  Transpose : Math  Operator=transpose
  Transpose1 : Math  Operator=transpose
  Vector Concatenate : Concatenate  NumInputs=3
  Out1 : Outport
  wires:
  Gain1/1 -> Plus/2  "10x1"
  Plus1/1 -> Matrix Multiply6/2  "10x3"
  Product3/1 -> Plus1/1  "10x3"
  Constant4/1 -> Product3/2
  Product2/1 -> Gain2/1  "10x1"
  Constant2/1 -> Gain1/1  "10x1"
  Constant6/1 -> Minus/2
  Constant3/1 -> Product2/1  "10x1"
  Product1/1 -> Matrix Multiply6/1  "10x3"
  Gain2/1 -> Plus/1  "10x1"
  " R_ B direction normalized"/1 -> Transpose/1  "3x1"
  Matrix Multiply3/1 -> Plus1/2  "10x3"
  Constant5/1 -> Minus/1
  Matrix Multiply6/1 -> Out1/1
  [Pos] -> Create Diagonal Matrix1/1  "10x1"
  Matrix Multiply1/1 -> Saturation1/1  "10x1"
  Constant12/1 -> Matrix Multiply1/1
  Minus/1 -> Matrix Multiply3/1  "10x1"
  Transpose/1 -> Matrix Multiply3/2  "1x3"
  Saturation1/1 -> [Pos]
  [Pos] -> Product2/2  "10x1"
  Plus/1 -> Create Diagonal Matrix/1
  Constant13/1 -> Vector Concatenate/3
  Constant10/1 -> Vector Concatenate/1
  Constant11/1 -> Vector Concatenate/2
  Vector Concatenate/1 -> Transpose1/1
  Create Diagonal Matrix/1 -> Product3/1  "10x10"
  Transpose1/1 -> Product5/2  "1x3"
  Constant8/1 -> Product5/1  "10x1"
  Product5/1 -> Product4/2  "10x3"
  Create Diagonal Matrix1/1 -> Product1/1  "10x3"
  Product4/1 -> Product1/2
  S/C direction normalized1/1 -> Matrix Multiply1/2  "3x1"
  Constant7/1 -> Divide/1
  Divide/1 -> Square/1
  Constant1/1 -> Product/1
  Square/1 -> Product/2
  Constant/1 -> Product/3
  In2/1 -> Product/4
  Product/1 -> Divide1/1
  Constant9/1 -> Divide1/2
  Divide1/1 -> [P_alb]
  [P_alb] -> Product4/1  "1x1"
  Sqrt/1 -> Divide/2
  R_B/1 -> Dot Product/1, Dot Product/2  "3x1"
  Dot Product/1 -> Sqrt/1

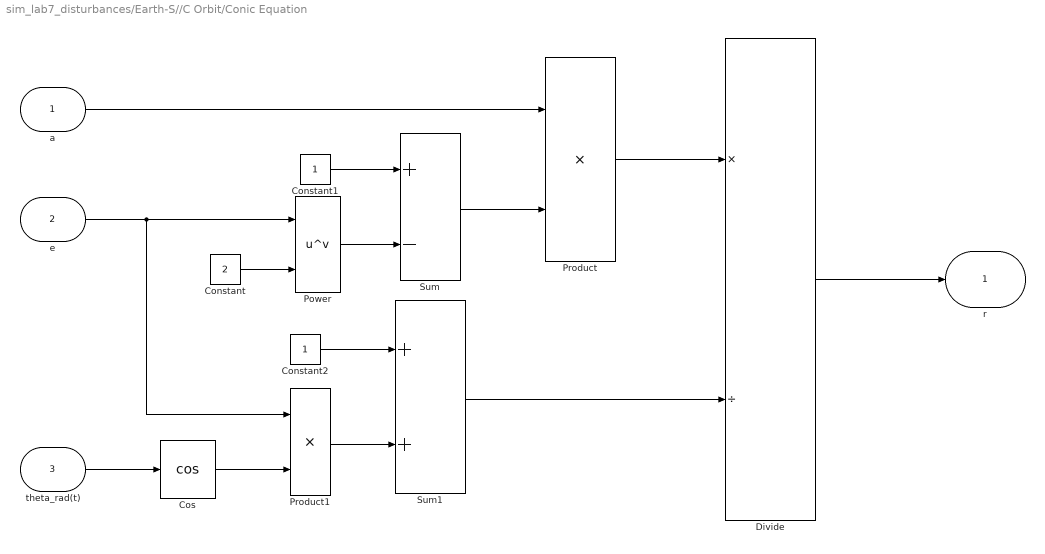
== system sim_lab7_disturbances/Earth-S//C Orbit/Conic Equation ==
  a : Inport
  e : Inport  Port=2
  theta_rad(t) : Inport  Port=3
  Constant : Constant  Value=2
  Constant1 : Constant
  Constant2 : Constant
  Cos : Trigonometry  Operator=cos
  Divide : Product  Inputs=*/
  Power : Math  Operator=pow
  Product : Product
  Product1 : Product
  Sum : Sum  Inputs=+-
  Sum1 : Sum
  r : Outport
  wires:
  a/1 -> Product/1
  e/1 -> Product1/1, Power/1
  Constant/1 -> Power/2
  Power/1 -> Sum/2
  Constant1/1 -> Sum/1
  Sum/1 -> Product/2
  Product/1 -> Divide/1
  Divide/1 -> r/1
  Constant2/1 -> Sum1/1
  theta_rad(t)/1 -> Cos/1
  Cos/1 -> Product1/2
  Product1/1 -> Sum1/2
  Sum1/1 -> Divide/2

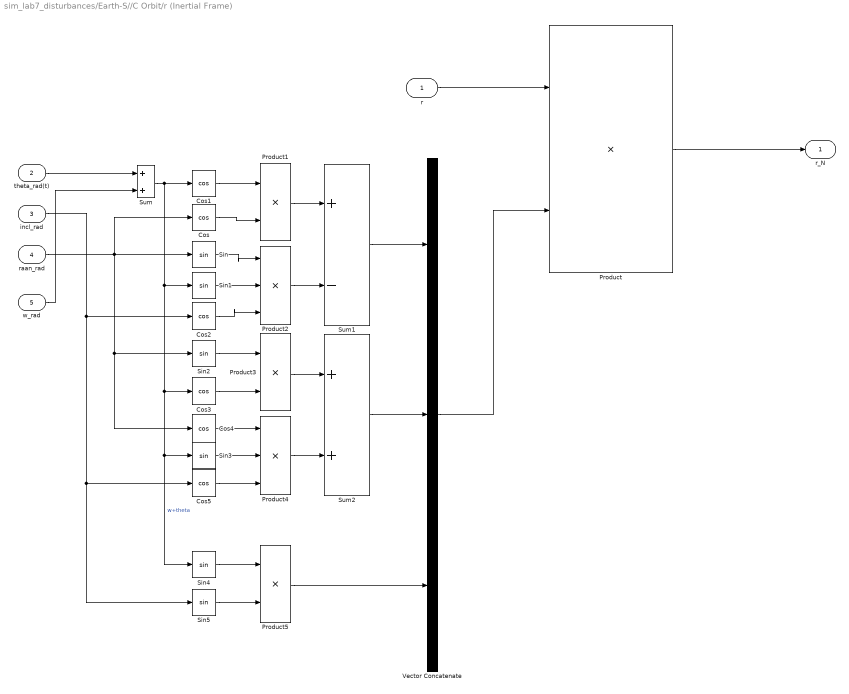
== system sim_lab7_disturbances/Earth-S//C Orbit/r (Inertial Frame) ==
  r : Inport
  theta_rad(t) : Inport  Port=2
  incl_rad : Inport  Port=3
  raan_rad : Inport  Port=4
  w_rad : Inport  Port=5
  Cos{,1..5} (6 alike) : Trigonometry  Operator=cos
  Product{,1,3,5} (4 alike) : Product
  Product2 : Product  Inputs=3
  Product4 : Product  Inputs=3
  Sin{,1..5} (6 alike) : Trigonometry
  Sum : Sum
  Sum1 : Sum  Inputs=+-
  Sum2 : Sum
  Vector Concatenate : Concatenate  NumInputs=3
  r_N : Outport
  wires:
  r/1 -> Product/1
  raan_rad/1 -> Cos/1, Cos4/1, Sin2/1, Sin/1
  w_rad/1 -> Sum/2
  Cos/1 -> Product1/2
  theta_rad(t)/1 -> Sum/1
  Sum/1 -> Sin4/1, Sin3/1, Cos3/1, Sin1/1, Cos1/1  "w+theta"
  Cos1/1 -> Product1/1
  Product1/1 -> Sum1/1
  Product2/1 -> Sum1/2
  Sin/1 -> Product2/1
  Sin1/1 -> Product2/2
  Cos2/1 -> Product2/3
  incl_rad/1 -> Cos5/1, Sin5/1, Cos2/1
  Sum1/1 -> Vector Concatenate/1
  Sum2/1 -> Vector Concatenate/2
  Sin2/1 -> Product3/1
  Cos3/1 -> Product3/2
  Product3/1 -> Sum2/1
  Product4/1 -> Sum2/2
  Cos4/1 -> Product4/1
  Sin3/1 -> Product4/2
  Cos5/1 -> Product4/3
  Sin4/1 -> Product5/1
  Sin5/1 -> Product5/2
  Product5/1 -> Vector Concatenate/3
  Vector Concatenate/1 -> Product/2
  Product/1 -> r_N/1

== system sim_lab7_disturbances/Magnetic Torque/B_N (IGRF Gauss Model - Order N) ==
  r_S/C_N : Inport
  Clock : Clock
  Constant : Constant  Value=Re
  Constant1 : Constant  Value=w_E
  MATLAB Function : MATLAB Function  TreatAsAtomicUnit=on
  Out1 : Outport
  wires:
  r_S/C_N/1 -> MATLAB Function/1(r_ECI)
  Clock/1 -> MATLAB Function/2(t)
  Constant/1 -> MATLAB Function/3(Re)
  Constant1/1 -> MATLAB Function/4(w_E)

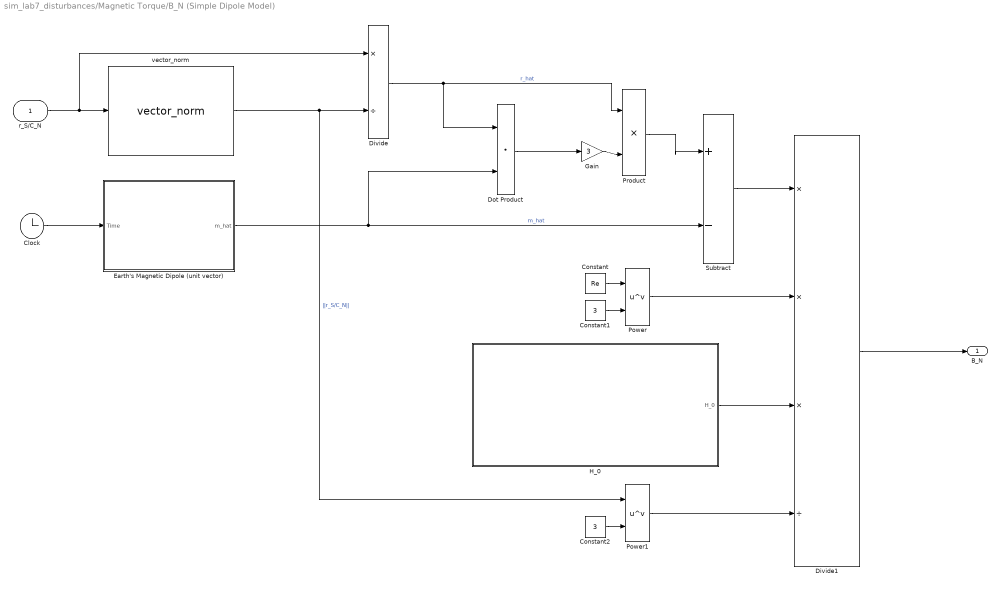
== system sim_lab7_disturbances/Magnetic Torque/B_N (Simple Dipole Model) ==
  r_S/C_N : Inport
  Clock : Clock
  Constant : Constant  Value=Re
  Constant1 : Constant  Value=3
  Constant2 : Constant  Value=3
  Divide : Product  Inputs=*/
  Divide1 : Product  Inputs=***/
  Dot Product : DotProduct  OutDataTypeStr=Inherit: Inherit via internal rule
  Earth's Magnetic Dipole (unit vector) : Subsystem
  Gain : Gain  Gain=3
  H_0 : Subsystem
  Power : Math  Operator=pow
  Power1 : Math  Operator=pow
  Product : Product
  Subtract : Sum  Inputs=+-
  vector_norm : LIBRARY_SAD/vector_norm  SystemSampleTime=-1  VariantActivationTime=update diagram  EmptyChoice=off  PassThrough=off  PassThroughVariantControl=(default)  EmptyChoiceVariantControl=(default)  AllowFlexibleInterface=on  Latency=0  AutoFrameSizeCalculation=off
  B_N : Outport
  wires:
  Clock/1 -> Earth's Magnetic Dipole (unit vector)/1(Time)
  Constant/1 -> Power/1
  Product/1 -> Subtract/1
  Divide/1 -> Dot Product/1, Product/1  "r_hat"
  Constant1/1 -> Power/2
  Divide1/1 -> B_N/1
  Subtract/1 -> Divide1/1
  Power/1 -> Divide1/2
  Power1/1 -> Divide1/4
  H_0/1(H_0) -> Divide1/3
  Dot Product/1 -> Gain/1
  Constant2/1 -> Power1/2
  vector_norm/1 -> Divide/2, Power1/1  "||r_S/C_N||"
  r_S/C_N/1 -> Divide/1, vector_norm/1
  Gain/1 -> Product/2
  Earth's Magnetic Dipole (unit vector)/1(m_hat) -> Subtract/2, Dot Product/2  "m_hat"

== system sim_lab7_disturbances/Solar Radiation Torque (SRP)/Body 1 ==
  Constant : Constant  Value=SRP.body1.A
  Constant1 : Constant  Value=SRP.body1.N_hat
  Constant2 : Constant  Value=SRP.body1.rho_s
  Constant3 : Constant  Value=SRP.body1.rho_d
  A_i : Outport
  N_B_hat_i : Outport  Port=2
  rho_s_i : Outport  Port=3
  rho_d_i : Outport  Port=4
  wires:
  Constant/1 -> A_i/1
  Constant1/1 -> N_B_hat_i/1
  Constant2/1 -> rho_s_i/1
  Constant3/1 -> rho_d_i/1

== system sim_lab7_disturbances/Solar Radiation Torque (SRP)/Body 2 ==
  Constant : Constant  Value=SRP.body2.A
  Constant1 : Constant  Value=SRP.body2.N_hat
  Constant2 : Constant  Value=SRP.body2.rho_s
  Constant3 : Constant  Value=SRP.body2.rho_d
  A_i : Outport
  N_B_hat_i : Outport  Port=2
  rho_s_i : Outport  Port=3
  rho_d_i : Outport  Port=4
  wires:
  Constant3/1 -> rho_d_i/1
  Constant2/1 -> rho_s_i/1
  Constant1/1 -> N_B_hat_i/1
  Constant/1 -> A_i/1

== system sim_lab7_disturbances/Solar Radiation Torque (SRP)/Body 3 ==
  Constant : Constant  Value=SRP.body3.A
  Constant1 : Constant  Value=SRP.body3.N_hat
  Constant2 : Constant  Value=SRP.body3.rho_s
  Constant3 : Constant  Value=SRP.body3.rho_d
  A_i : Outport
  N_B_hat_i : Outport  Port=2
  rho_s_i : Outport  Port=3
  rho_d_i : Outport  Port=4
  wires:
  Constant/1 -> A_i/1
  Constant1/1 -> N_B_hat_i/1
  Constant2/1 -> rho_s_i/1
  Constant3/1 -> rho_d_i/1

== system sim_lab7_disturbances/Solar Radiation Torque (SRP)/Body 4 ==
  Constant : Constant  Value=SRP.body4.A
  Constant1 : Constant  Value=SRP.body4.N_hat
  Constant2 : Constant  Value=SRP.body4.rho_s
  Constant3 : Constant  Value=SRP.body4.rho_d
  A_i : Outport
  N_B_hat_i : Outport  Port=2
  rho_s_i : Outport  Port=3
  rho_d_i : Outport  Port=4
  wires:
  Constant3/1 -> rho_d_i/1
  Constant2/1 -> rho_s_i/1
  Constant1/1 -> N_B_hat_i/1
  Constant/1 -> A_i/1

== system sim_lab7_disturbances/Solar Radiation Torque (SRP)/Body 5 ==
  Constant : Constant  Value=SRP.body5.A
  Constant1 : Constant  Value=SRP.body5.N_hat
  Constant2 : Constant  Value=SRP.body5.rho_s
  Constant3 : Constant  Value=SRP.body5.rho_d
  A_i : Outport
  N_B_hat_i : Outport  Port=2
  rho_s_i : Outport  Port=3
  rho_d_i : Outport  Port=4
  wires:
  Constant/1 -> A_i/1
  Constant1/1 -> N_B_hat_i/1
  Constant2/1 -> rho_s_i/1
  Constant3/1 -> rho_d_i/1

== system sim_lab7_disturbances/Solar Radiation Torque (SRP)/Body 6 ==
  Constant : Constant  Value=SRP.body6.A
  Constant1 : Constant  Value=SRP.body6.N_hat
  Constant2 : Constant  Value=SRP.body6.rho_s
  Constant3 : Constant  Value=SRP.body6.rho_d
  A_i : Outport
  N_B_hat_i : Outport  Port=2
  rho_s_i : Outport  Port=3
  rho_d_i : Outport  Port=4
  wires:
  Constant3/1 -> rho_d_i/1
  Constant2/1 -> rho_s_i/1
  Constant1/1 -> N_B_hat_i/1
  Constant/1 -> A_i/1

== system sim_lab7_disturbances/Solar Radiation Torque (SRP)/Panel 1 ==
  Constant : Constant  Value=SRP.panel1.A
  Constant1 : Constant  Value=SRP.panel1.N_hat
  Constant2 : Constant  Value=SRP.panel1.rho_s
  Constant3 : Constant  Value=SRP.panel1.rho_d
  A_i : Outport
  N_B_hat_i : Outport  Port=2
  rho_s_i : Outport  Port=3
  rho_d_i : Outport  Port=4
  wires:
  Constant/1 -> A_i/1
  Constant1/1 -> N_B_hat_i/1
  Constant2/1 -> rho_s_i/1
  Constant3/1 -> rho_d_i/1

== system sim_lab7_disturbances/Solar Radiation Torque (SRP)/Panel 2 ==
  Constant : Constant  Value=SRP.panel2.A
  Constant1 : Constant  Value=SRP.panel2.N_hat
  Constant2 : Constant  Value=SRP.panel2.rho_s
  Constant3 : Constant  Value=SRP.panel2.rho_d
  A_i : Outport
  N_B_hat_i : Outport  Port=2
  rho_s_i : Outport  Port=3
  rho_d_i : Outport  Port=4
  wires:
  Constant3/1 -> rho_d_i/1
  Constant2/1 -> rho_s_i/1
  Constant1/1 -> N_B_hat_i/1
  Constant/1 -> A_i/1

== system sim_lab7_disturbances/Solar Radiation Torque (SRP)/Panel 3 ==
  Constant : Constant  Value=SRP.panel3.A
  Constant1 : Constant  Value=SRP.panel3.N_hat
  Constant2 : Constant  Value=SRP.panel3.rho_s
  Constant3 : Constant  Value=SRP.panel3.rho_d
  A_i : Outport
  N_B_hat_i : Outport  Port=2
  rho_s_i : Outport  Port=3
  rho_d_i : Outport  Port=4
  wires:
  Constant/1 -> A_i/1
  Constant1/1 -> N_B_hat_i/1
  Constant2/1 -> rho_s_i/1
  Constant3/1 -> rho_d_i/1

== system sim_lab7_disturbances/Solar Radiation Torque (SRP)/Panel 4 ==
  Constant : Constant  Value=SRP.panel4.A
  Constant1 : Constant  Value=SRP.panel4.N_hat
  Constant2 : Constant  Value=SRP.panel4.rho_s
  Constant3 : Constant  Value=SRP.panel4.rho_d
  A_i : Outport
  N_B_hat_i : Outport  Port=2
  rho_s_i : Outport  Port=3
  rho_d_i : Outport  Port=4
  wires:
  Constant3/1 -> rho_d_i/1
  Constant2/1 -> rho_s_i/1
  Constant1/1 -> N_B_hat_i/1
  Constant/1 -> A_i/1

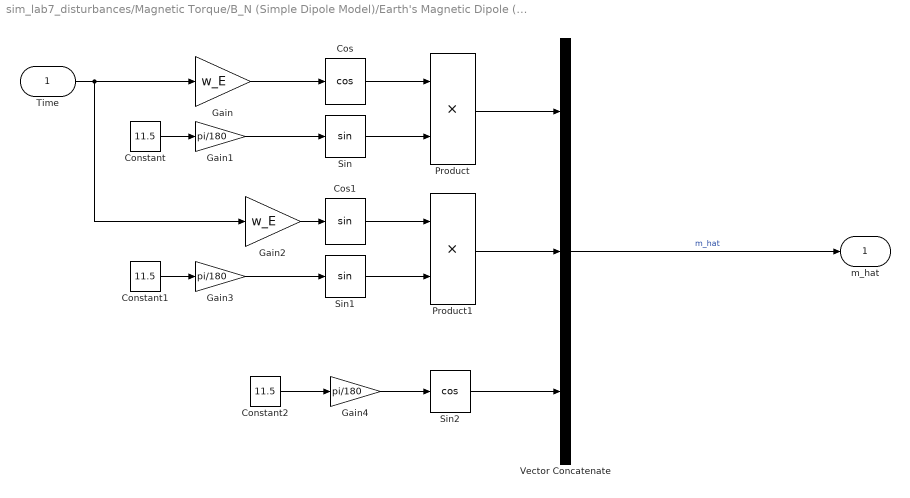
== system sim_lab7_disturbances/Magnetic Torque/B_N (Simple Dipole Model)/Earth's Magnetic Dipole (unit vector) ==
  Time : Inport
  Constant : Constant  Value=11.5
  Constant1 : Constant  Value=11.5
  Constant2 : Constant  Value=11.5
  Cos : Trigonometry  Operator=cos
  Cos1 : Trigonometry
  Gain : Gain  Gain=w_E
  Gain1 : Gain  Gain=pi/180
  Gain2 : Gain  Gain=w_E
  Gain3 : Gain  Gain=pi/180
  Gain4 : Gain  Gain=pi/180
  Product : Product
  Product1 : Product
  Sin : Trigonometry
  Sin1 : Trigonometry
  Sin2 : Trigonometry  Operator=cos
  Vector Concatenate : Concatenate  NumInputs=3
  m_hat : Outport
  wires:
  Gain/1 -> Cos/1
  Cos/1 -> Product/1
  Sin/1 -> Product/2
  Constant/1 -> Gain1/1
  Gain1/1 -> Sin/1
  Product/1 -> Vector Concatenate/1
  Product1/1 -> Vector Concatenate/2
  Cos1/1 -> Product1/1
  Gain2/1 -> Cos1/1
  Time/1 -> Gain2/1, Gain/1
  Constant2/1 -> Gain4/1
  Gain4/1 -> Sin2/1
  Sin2/1 -> Vector Concatenate/3
  Vector Concatenate/1 -> m_hat/1  "m_hat"
  Gain3/1 -> Sin1/1
  Constant1/1 -> Gain3/1
  Sin1/1 -> Product1/2

== system sim_lab7_disturbances/Magnetic Torque/B_N (Simple Dipole Model)/H_0 ==
  Constant1 : Constant  Value=2
  Constant2 : Constant  Value=2
  Constant3 : Constant  Value=g0_1
  Constant4 : Constant  Value=g1_1
  Constant5 : Constant  Value=2
  Constant6 : Constant  Value=h1_1
  Power : Math  Operator=pow
  Power1 : Math  Operator=pow
  Power2 : Math  Operator=pow
  Sqrt : Sqrt
  Sum : Sum  Inputs=+++
  H_0 : Outport
  wires:
  Constant3/1 -> Power/1
  Power2/1 -> Sum/3
  Power1/1 -> Sum/2
  Sqrt/1 -> H_0/1
  Power/1 -> Sum/1
  Sum/1 -> Sqrt/1
  Constant1/1 -> Power/2
  Constant2/1 -> Power1/2
  Constant4/1 -> Power1/1
  Constant6/1 -> Power2/1
  Constant5/1 -> Power2/2

== matlab function sim_lab7_disturbances/Magnetic Torque/B_N (IGRF Gauss Model - Order N)/MATLAB Function ==
  data: r_ECI input; B_N output; t input; Re input; w_E input
function B_N = magnetic_field_ECI(r_ECI, t, Re, w_E)
% Earth's Magnetic Field vector in Inertial Frame (ECI) 
% INPUT:
%   r_ECI : position vector [km] (ECI)
%   t     : time [s] (from reference epoch, i.e. J2000)
%   Re : equatorial radius of the Earth      [km]
%   w_E : averaged angular velocity of the Earth [rad/s]
% OUTPUT:
%   B_ECI : magnetic field [T] (ECI)

% -------------------------------------------------

% Greenwich Right Ascension (Greenwich Sidereal Time)
ra_GST = mod(w_E * t, 2*pi);

% Rotation Matrix ECI -> ECEF
Rz = [cos(ra_GST)  sin(ra_GST)  0;
     -sin(ra_GST)  cos(ra_GST)  0;
      0               0         1];

% Position vector in ECEF Frame 
r_ECEF = Rz * r_ECI;

% Magnetic Field in IGRF Model (up to Nmax order approximation)
Nmax = 9;
B_ECEF = igrf_gauss_model_ECEF(r_ECEF, Nmax);

% Converting back B_ECEF -> B_ECI (B_N)
B_N = Rz' * B_ECEF;
end


function B_ECEF = igrf_gauss_model_ECEF(r_ECEF, Nmax)
% Magnetic Field in ECEF based on Gauss Model with
% Schmidt-quasi-normalized/Legendre Polynomials

% Coefficients (IGRF-13, epoch 2020.0, nT)
g = zeros(Nmax+1,Nmax+1);
h = zeros(Nmax+1,Nmax+1);
g(1,1) = -29404.8; h(1,1) = 0;
g(1,2) = -1450.9;  h(1,2) = 4652.5;
g(2,1) = -2500.0;  h(2,1) = 0;
g(2,2) = 2982.0;   h(2,2) = -2991.6;
g(2,3) = 1676.8;   h(2,3) = -734.8;

% Coordinate sferiche
x = r_ECEF(1); y = r_ECEF(2); z = r_ECEF(3);
r = norm(r_ECEF);
theta = acos(z/r);     % colatitudine (0 = Nord)
phi = atan2(y,x);

% Polinomi di Legendre normalizzati
P = legendre_matrix(Nmax, cos(theta));

Br = 0; 
Btheta = 0; 
Bphi = 0;

for n = 1:Nmax
    for m = 0:n
        gnm = g(n,m+1);
        hnm = h(n,m+1);
        r_ratio = (Re/r)^(n+2);
        cosmf = cos(m*phi);
        sinmf = sin(m*phi);
        Vnm = gnm*cosmf + hnm*sinmf;

        Br = Br + (n+1)*r_ratio * Vnm * P(n+1,m+1);
        dP = dPnm_dtheta(n,m,theta);
        Btheta = Btheta - r_ratio * Vnm * dP;
        Bphi = Bphi + r_ratio * m * (hnm*cosmf - gnm*sinmf) * P(n+1,m+1);
    end
end

% Conversion in ECEF Frame
B_r = -Br;
B_theta = -Btheta / r;
B_phi = -Bphi / (r * sin(theta));
B_ECEF = spherical_to_cartesian(B_r,B_theta,B_phi,theta,phi) * 1e-9; % T
end


% ------------ AUXILIARY FUNCTIONS  ------------------------

function P = legendre_matrix(N, x)
    P = zeros(N+1,N+1);
    for n=0:N
        P(n+1,1:n+1) = legendre(n,x,'sch');
    end
end

function dP = dPnm_dtheta(n,m,theta)
    dP = (m*cos(theta)*legendreP(n,m,cos(theta)) - (n+m)*legendreP(n-1,m,cos(theta)))/sin(theta);
end

function Bxyz = spherical_to_cartesian(Br,Bt,Bp,theta,phi)
    Bx = Br*sin(theta)*cos(phi) + Bt*cos(theta)*cos(phi) - Bp*sin(phi);
    By = Br*sin(theta)*sin(phi) + Bt*cos(theta)*sin(phi) + Bp*cos(phi);
    Bz = Br*cos(theta) - Bt*sin(theta);
    Bxyz = [Bx; By; Bz];
end

function [ra,dec] = ra_and_dec_from_r(r)
%RA_AND_DEC_FROM_R This function computes the RA and declination (in Earth
%Equatorial Inertial Frame) given the vector r

% INPUTS: r : position vector  in EC/EQ

% OUTPUTS : ra: Right Ascension in Earth Centered Equatorial Inertial Frame
%               [deg]
%           dec: Declination in Earth Centred Equatorial Inertial frame [deg]

% Direction cosine
n = r(3)/norm(r);

% Computing declination
dec = asind(n);

% Computing right ascension
ra = atan2d(r(2),r(1));

end
